simulink model "Quadcopter_nonlinear_LQIDG"  (R2020a)
settings: Solver=ode4  StartTime=0.0  StopTime=15  FixedStep=0.02  RelTol=1e-3
InitFcn:
  | Roll_OpenLoop_LQIDG_solver;
  | Pitch_OpenLoop_LQIDG_solver;
  | Yaw_OpenLoop_LQIDG_solver;
values from neighbouring files (symbols this model uses):
  A1 = 6.52172868745337    (= 6.52172868745)    [roll_pitch_yaw_parameter_estimation.m]
  A2 = -1.56517460219627    (= -1.5651746022)    [roll_pitch_yaw_parameter_estimation.m]
  A3 = 5.18692283683343e-05    (= 5.18692283683e-05)    [roll_pitch_yaw_parameter_estimation.m]
  A4 = 0.00249993776857667    (= 0.00249993776858)    [roll_pitch_yaw_parameter_estimation.m]
  A5 = -0.259645819519501    (= -0.25964581952)    [roll_pitch_yaw_parameter_estimation.m]
  A6 = 1.37409031322133    (= 1.37409031322)    [roll_pitch_yaw_parameter_estimation.m]
  B1 = 4.36026813860301    (= 4.3602681386)    [roll_pitch_yaw_parameter_estimation.m]
  B2 = 1.57068812881144    (= 1.57068812881)    [roll_pitch_yaw_parameter_estimation.m]
  B3 = 6.9083e-05    [roll_pitch_yaw_parameter_estimation.m]
  B4 = -0.00274841569825112    (= -0.00274841569825)    [roll_pitch_yaw_parameter_estimation.m]
  B5 = 0.595980110229882    (= 0.59598011023)    [roll_pitch_yaw_parameter_estimation.m]
  B6 = 4.42876359313229    (= 4.42876359313)    [roll_pitch_yaw_parameter_estimation.m]
  C1 = 0.0856557051952501    (= 0.0856557051953)    [roll_pitch_yaw_parameter_estimation.m]
  C2 = 1.26915503141054e-06    (= 1.26915503141e-06)    [roll_pitch_yaw_parameter_estimation.m]
  C3 = 0.178562738125068    (= 0.178562738125)    [roll_pitch_yaw_parameter_estimation.m]
  LQIDG_openloop_roll = (R1_inv * B' * p1)    [Roll_OpenLoop_LQIDG_solver.m]
undefined symbols (not defined in the file or in its folder): DiscIntNeverNeededParam, LQIDG_openloop_pitch, LQIDG_openloop_yaw, magnitude
libraries: simulink x1, simulink_extras x1
settings Model: Creator=Ali  LastModifiedBy=Ali

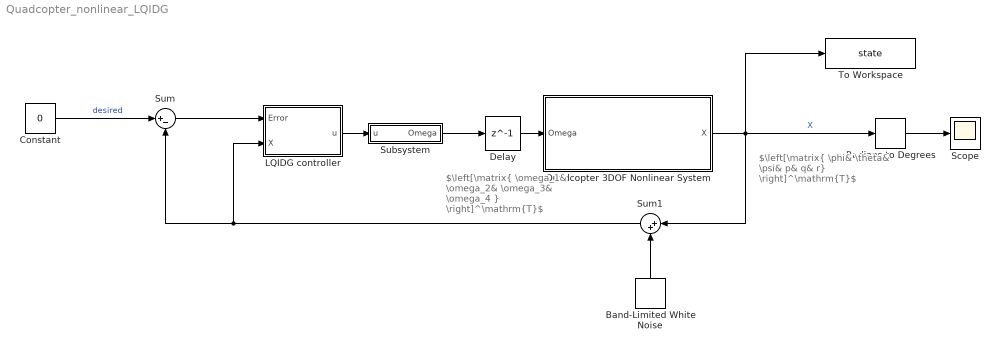
== system Quadcopter_nonlinear_LQIDG ==
  note: $\left[\matrix{ \omega_1& \omega_2& \omega_3& \omega_4 } \right]^\mathrm{T}$
  note: $\left[\matrix{ \phi& \theta& \psi& p& q& r} \right]^\mathrm{T}$
  Band-Limited White Noise : simulink/Sources/Band-Limited White Noise  Cov=[0.00001]  Ts=0.02  seed=[23341]
  Constant : Constant  Value=0
  Delay : Delay  DelayLength=1
  LQIDG controller : Subsystem
  Quadcopter 3DOF Nonlinear System : Subsystem  TreatAsAtomicUnit=on
      mask Display: image('quad1.png'); % Use "Edit Image" on toolstrip to change.
  Radians to Degrees : simulink_extras/Transformations/Radians to Degrees
  Scope : Scope
  Subsystem : Subsystem
  Sum : Sum  Inputs=|+-
  Sum1 : Sum  Inputs=|++
  To Workspace : ToWorkspace  VariableName=state  SampleTime=-1
  wires:
  Subsystem/1(Omega) -> Delay/1
  LQIDG controller/1(u) -> Subsystem/1(u)
  Sum/1 -> LQIDG controller/1(Error)
  Constant/1 -> Sum/1  "desired"
  Quadcopter 3DOF Nonlinear System/1(X) -> To Workspace/1, Sum1/1, Radians to Degrees/1  "X"
  Delay/1 -> Quadcopter 3DOF Nonlinear System/1(Omega)
  Radians to Degrees/1 -> Scope/1
  Sum1/1 -> LQIDG controller/2(X), Sum/2
  Band-Limited White Noise/1 -> Sum1/2

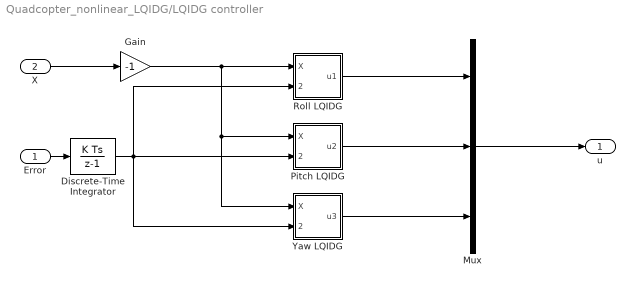
== system Quadcopter_nonlinear_LQIDG/LQIDG controller ==
  Error : Inport
  X : Inport  Port=2
  Discrete-Time Integrator : DiscreteIntegrator  SampleTime=-1  UpperSaturationLimit=2  LowerSaturationLimit=-2  ICPrevOutput=DiscIntNeverNeededParam  ICPrevScaledInput=DiscIntNeverNeededParam
  Gain : Gain  Gain=-1
  Mux : Mux  Inputs=3
  Pitch LQIDG : Subsystem
  Roll LQIDG : Subsystem
  Yaw LQIDG : Subsystem
  u : Outport
  wires:
  X/1 -> Gain/1
  Gain/1 -> Yaw LQIDG/1(X), Pitch LQIDG/1(X), Roll LQIDG/1(X)
  Error/1 -> Discrete-Time Integrator/1
  Roll LQIDG/1(u1) -> Mux/1
  Pitch LQIDG/1(u2) -> Mux/2
  Yaw LQIDG/1(u3) -> Mux/3
  Mux/1 -> u/1
  Discrete-Time Integrator/1 -> Roll LQIDG/2(Error), Yaw LQIDG/2(Error), Pitch LQIDG/2(Error)

== system Quadcopter_nonlinear_LQIDG/Quadcopter 3DOF Nonlinear System ==
  note: $\dot X$
  note: $\left[\matrix{ \dot\phi& \dot\theta& \dot\psi& \dot p& \dot q& \dot r} \right]^\mathrm{T}$
  note: $\left[\matrix{ \phi& \theta& \psi& p& q& r} \right]^\mathrm{T}$
  Omega : Inport
  Integrator : Integrator  InitialCondition=[-0.5, -1, 1, 0, 0, 0]
  Quad System : Subsystem
  Subsystem : Subsystem
  X : Outport
  wires:
  Integrator/1 -> Quad System/1(X), X/1  "X"
  Quad System/1(dot(X)) -> Integrator/1  "dot(X)"
  Omega/1 -> Subsystem/1(motor command)
  Subsystem/1(motor output) -> Quad System/2(Omega)

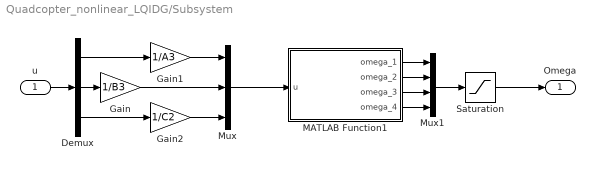
== system Quadcopter_nonlinear_LQIDG/Subsystem ==
  u : Inport
  Demux : Demux  Outputs=3
  Gain : Gain  Gain=1/B3
  Gain1 : Gain  Gain=1/A3
  Gain2 : Gain  Gain=1/C2
  MATLAB Function1 : MATLAB Function  TreatAsAtomicUnit=on
  Mux : Mux  Inputs=3
  Mux1 : Mux
  Saturation : Saturate  UpperLimit=6000/60*2*pi  LowerLimit=1300/60*2*pi
  Omega : Outport
  wires:
  MATLAB Function1/1(omega_1) -> Mux1/1
  MATLAB Function1/2(omega_2) -> Mux1/2
  MATLAB Function1/4(omega_4) -> Mux1/4
  MATLAB Function1/3(omega_3) -> Mux1/3
  Mux1/1 -> Saturation/1
  Mux/1 -> MATLAB Function1/1(u)
  Gain/1 -> Mux/2
  Gain1/1 -> Mux/1
  u/1 -> Demux/1
  Demux/2 -> Gain/1
  Demux/1 -> Gain1/1
  Demux/3 -> Gain2/1
  Gain2/1 -> Mux/3
  Saturation/1 -> Omega/1

== system Quadcopter_nonlinear_LQIDG/LQIDG controller/Pitch LQIDG ==
  X : Inport
  Error : Inport  Port=2
  Constant : Constant  Value=LQIDG_openloop_pitch
  Mux : Mux  Inputs=2
  Product : Product  Multiplication=Matrix(*)
  Selector : Selector  InputPortWidth=6  IndexOptions=Index vector (dialog)  Indices=[2 5]  OutputSizes=1
  Selector1 : Selector  InputPortWidth=6  IndexOptions=Index vector (dialog)  Indices=[2 5]  OutputSizes=1
  u2 : Outport
  wires:
  Product/1 -> u2/1
  Constant/1 -> Product/2
  Selector1/1 -> Mux/2
  Selector/1 -> Mux/1
  Error/1 -> Selector1/1
  X/1 -> Selector/1
  Mux/1 -> Product/1

== system Quadcopter_nonlinear_LQIDG/LQIDG controller/Roll LQIDG ==
  X : Inport
  Error : Inport  Port=2
  Constant : Constant  Value=LQIDG_openloop_roll
  Mux : Mux  Inputs=2
  Product : Product  Multiplication=Matrix(*)
  Selector : Selector  InputPortWidth=6  IndexOptions=Index vector (dialog)  Indices=[1 4]  OutputSizes=1
  Selector1 : Selector  InputPortWidth=6  IndexOptions=Index vector (dialog)  Indices=[1 4]  OutputSizes=1
  u1 : Outport
  wires:
  Product/1 -> u1/1
  Constant/1 -> Product/2
  X/1 -> Selector/1
  Error/1 -> Selector1/1
  Mux/1 -> Product/1
  Selector/1 -> Mux/1
  Selector1/1 -> Mux/2

== system Quadcopter_nonlinear_LQIDG/LQIDG controller/Yaw LQIDG ==
  X : Inport
  Error : Inport  Port=2
  Constant : Constant  Value=LQIDG_openloop_yaw
  Mux : Mux  Inputs=2
  Product : Product  Multiplication=Matrix(*)
  Selector : Selector  InputPortWidth=6  IndexOptions=Index vector (dialog)  Indices=[3 6]  OutputSizes=1
  Selector1 : Selector  InputPortWidth=6  IndexOptions=Index vector (dialog)  Indices=[3 6]  OutputSizes=1
  u3 : Outport
  wires:
  Product/1 -> u3/1
  Constant/1 -> Product/2
  Mux/1 -> Product/1
  Selector1/1 -> Mux/2
  Error/1 -> Selector1/1
  X/1 -> Selector/1
  Selector/1 -> Mux/1

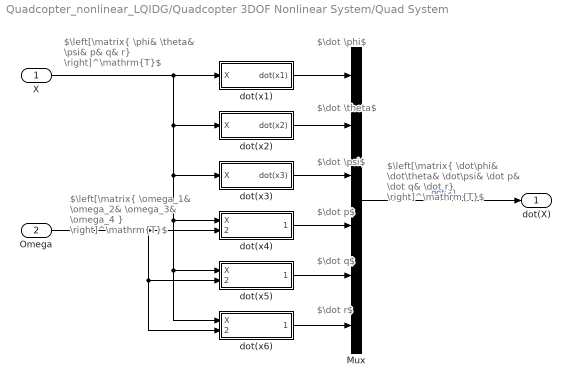
== system Quadcopter_nonlinear_LQIDG/Quadcopter 3DOF Nonlinear System/Quad System ==
  note: $\dot \phi$
  note: $\left[\matrix{ \phi& \theta& \psi& p& q& r} \right]^\mathrm{T}$
  note: $\left[\matrix{ \omega_1& \omega_2& \omega_3& \omega_4 } \right]^\mathrm{T}$
  note: $\dot \theta$
  note: $\dot \psi$
  note: $\dot p$
  note: $\dot q$
  note: $\dot r$
  note: $\left[\matrix{ \dot\phi& \dot\theta& \dot\psi& \dot p& \dot q& \dot r} \right]^\mathrm{T}$
  X : Inport
  Omega : Inport  Port=2
  Mux : Mux  Inputs=6
  dot(x1) : Subsystem
  dot(x2) : Subsystem
  dot(x3) : Subsystem
  dot(x4) : Subsystem
  dot(x5) : Subsystem
  dot(x6) : Subsystem
  dot(X) : Outport
  wires:
  Mux/1 -> dot(X)/1  "dot(X)"
  X/1 -> dot(x6)/1(X), dot(x5)/1(X), dot(x4)/1(X), dot(x3)/1(X), dot(x2)/1(X), dot(x1)/1(X)
  Omega/1 -> dot(x6)/2(Omega), dot(x5)/2(Omega), dot(x4)/2(Omega)
  dot(x5)/1(dot(x5)) -> Mux/5
  dot(x2)/1(dot(x2)) -> Mux/2
  dot(x4)/1(dot(x4)) -> Mux/4
  dot(x3)/1(dot(x3)) -> Mux/3
  dot(x1)/1(dot(x1)) -> Mux/1
  dot(x6)/1(dot(x6)) -> Mux/6

== system Quadcopter_nonlinear_LQIDG/Quadcopter 3DOF Nonlinear System/Subsystem ==
  motor command : Inport
  For Each Subsystem : Subsystem  TreatAsAtomicUnit=on
  motor output : Outport
  wires:
  motor command/1 -> For Each Subsystem/1(Omega_c)
  For Each Subsystem/1(Omega_m) -> motor output/1

== system Quadcopter_nonlinear_LQIDG/Quadcopter 3DOF Nonlinear System/Quad System/dot(x1) ==
  X : Inport
  1 : Subsystem
  Add : Sum  Inputs=+++
  Subsystem : Subsystem
  Subsystem1 : Subsystem
  dot(x1) : Outport
  wires:
  X/1 -> Subsystem1/1(X), Subsystem/1(X), 1/1(X)  "X"
  Subsystem1/1(x4) -> Add/3
  Subsystem/1(x6cos(x1)tan(x2)) -> Add/2
  Add/1 -> dot(x1)/1
  1/1(x5sin(x1)tan(x2)) -> Add/1

== system Quadcopter_nonlinear_LQIDG/Quadcopter 3DOF Nonlinear System/Quad System/dot(x2) ==
  X : Inport
  1 : Subsystem
  Add : Sum  Inputs=+-
  Subsystem : Subsystem
  dot(x2) : Outport
  wires:
  X/1 -> Subsystem/1(X), 1/1(X)  "X"
  Subsystem/1(x6sin(x1)) -> Add/2
  Add/1 -> dot(x2)/1
  1/1(x5cos(x1)) -> Add/1

== system Quadcopter_nonlinear_LQIDG/Quadcopter 3DOF Nonlinear System/Quad System/dot(x3) ==
  X : Inport
  1 : Subsystem
  Add : Sum
  Product : Product
  Subsystem : Subsystem
  Subsystem1 : Subsystem
  dot(x3) : Outport
  wires:
  X/1 -> Subsystem1/1(X), Subsystem/1(X), 1/1(X)  "X"
  Subsystem/1(x6cos(x1)) -> Add/2
  1/1(x5sin(x1)) -> Add/1
  Product/1 -> dot(x3)/1
  Add/1 -> Product/1
  Subsystem1/1(sec(x2)) -> Product/2

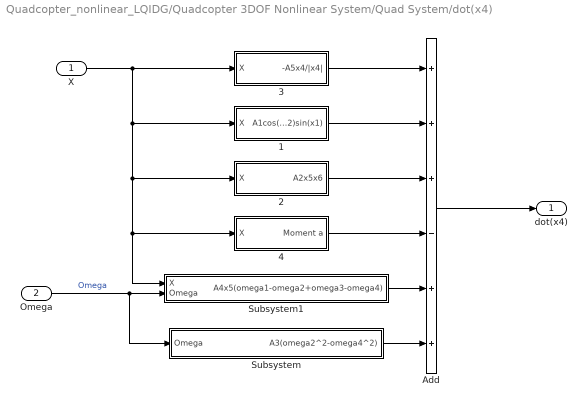
== system Quadcopter_nonlinear_LQIDG/Quadcopter 3DOF Nonlinear System/Quad System/dot(x4) ==
  X : Inport
  Omega : Inport  Port=2
  1 : Subsystem
  2 : Subsystem
  3 : Subsystem
  4 : Subsystem
  Add : Sum  Inputs=+++-++
  Subsystem : Subsystem
  Subsystem1 : Subsystem
  dot(x4) : Outport
  wires:
  X/1 -> 4/1(X), Subsystem1/1(X), 2/1(X), 1/1(X), 3/1(X)
  Omega/1 -> Subsystem/1(Omega), Subsystem1/2(Omega)  "Omega"
  Add/1 -> dot(x4)/1
  3/1("-A5x4/|x4| ") -> Add/1
  1/1(A1cos(x2)sin(x1)) -> Add/2
  2/1(A2x5x6) -> Add/3
  Subsystem1/1(A4x5(omega1-omega2+omega3-omega4)) -> Add/5
  Subsystem/1(A3(omega2^2-omega4^2)) -> Add/6
  4/1(Moment a) -> Add/4

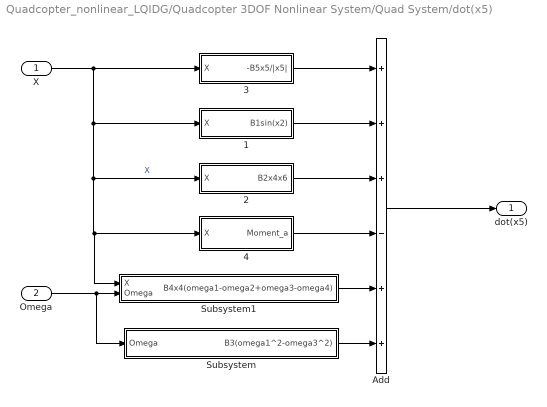
== system Quadcopter_nonlinear_LQIDG/Quadcopter 3DOF Nonlinear System/Quad System/dot(x5) ==
  X : Inport
  Omega : Inport  Port=2
  1 : Subsystem
  2 : Subsystem
  3 : Subsystem
  4 : Subsystem
  Add : Sum  Inputs=+++-++
  Subsystem : Subsystem
  Subsystem1 : Subsystem
  dot(x5) : Outport
  wires:
  Omega/1 -> Subsystem/1(Omega), Subsystem1/2(Omega)
  Add/1 -> dot(x5)/1
  3/1("-B5x5/|x5| ") -> Add/1
  1/1(B1sin(x2)) -> Add/2
  2/1(B2x4x6) -> Add/3
  Subsystem1/1(B4x4(omega1-omega2+omega3-omega4)) -> Add/5
  Subsystem/1(B3(omega1^2-omega3^2)) -> Add/6
  4/1(Moment_a) -> Add/4
  X/1 -> Subsystem1/1(X), 4/1(X), 2/1(X), 1/1(X), 3/1(X)  "X"

== system Quadcopter_nonlinear_LQIDG/Quadcopter 3DOF Nonlinear System/Quad System/dot(x6) ==
  X : Inport
  Omega : Inport  Port=2
  2 : Subsystem
  3 : Subsystem
  Add : Sum  Inputs=+++
  Subsystem : Subsystem
  dot(x6) : Outport
  wires:
  Omega/1 -> Subsystem/1(Omega)  "Omega"
  Add/1 -> dot(x6)/1
  3/1("-C3x6/|x6| ") -> Add/1
  2/1(C1x4x5) -> Add/2
  Subsystem/1(C2(omega1^2-omega2^2+omega3^2-omega4^2)) -> Add/3
  X/1 -> 2/1(X), 3/1(X)  "X"

== system Quadcopter_nonlinear_LQIDG/Quadcopter 3DOF Nonlinear System/Subsystem/For Each Subsystem ==
  Omega_c : Inport  Partition=on  PartitionDimension=1  PartitionWidth=1  PartitionOffset=0
  For Each : ForEach  DisableCoverage=on
  Transfer Fcn : TransferFcn  Denominator=[0.15 1]
  Omega_m : Outport  ConcatenationDimension=1
  wires:
  Omega_c/1 -> Transfer Fcn/1
  Transfer Fcn/1 -> Omega_m/1

== system Quadcopter_nonlinear_LQIDG/Quadcopter 3DOF Nonlinear System/Quad System/dot(x1)/1 ==
  X : Inport
  Demux : Demux  Outputs=6
  Subsystem : Subsystem
  Terminator : Terminator
  Terminator1 : Terminator
  Terminator2 : Terminator
  x5sin(x1)tan(x2) : Outport
  wires:
  Demux/2 -> Subsystem/2(x2)  "x2"
  Demux/4 -> Terminator1/1  "x4"
  X/1 -> Demux/1  "x"
  Demux/1 -> Subsystem/1(x1)  "x1"
  Demux/3 -> Terminator/1  "x3"
  Demux/6 -> Terminator2/1  "x6"
  Demux/5 -> Subsystem/3(x5)  "x5"
  Subsystem/1(x5sin(x1)tan(x2)) -> x5sin(x1)tan(x2)/1

== system Quadcopter_nonlinear_LQIDG/Quadcopter 3DOF Nonlinear System/Quad System/dot(x1)/Subsystem ==
  X : Inport
  Demux : Demux  Outputs=6
  Subsystem1 : Subsystem
  Terminator : Terminator
  Terminator1 : Terminator
  Terminator3 : Terminator
  x6cos(x1)tan(x2) : Outport
  wires:
  Demux/1 -> Subsystem1/1(x1)  "x1"
  Demux/3 -> Terminator/1  "x3"
  Demux/4 -> Terminator1/1  "x4"
  Demux/5 -> Terminator3/1  "x5"
  Demux/6 -> Subsystem1/3(x6)  "x6"
  Subsystem1/1(x6cos(x1)tan(x2)) -> x6cos(x1)tan(x2)/1  "x6cos(x1)tan(x2)"
  X/1 -> Demux/1  "X"
  Demux/2 -> Subsystem1/2(x2)  "x2"

== system Quadcopter_nonlinear_LQIDG/Quadcopter 3DOF Nonlinear System/Quad System/dot(x1)/Subsystem1 ==
  X : Inport
  Demux : Demux  Outputs=6
  Terminator{,2..5} (5 alike) : Terminator
  x4 : Outport
  wires:
  Demux/6 -> Terminator5/1  "x6"
  X/1 -> Demux/1
  Demux/3 -> Terminator/1  "x3"
  Demux/1 -> Terminator4/1  "x1"
  Demux/2 -> Terminator2/1  "x2"
  Demux/5 -> Terminator3/1  "x5"
  Demux/4 -> x4/1  "x4"

== system Quadcopter_nonlinear_LQIDG/Quadcopter 3DOF Nonlinear System/Quad System/dot(x2)/1 ==
  X : Inport
  Demux : Demux  Outputs=6
  Subsystem : Subsystem
  Terminator{,1..3} (4 alike) : Terminator
  x5cos(x1) : Outport
  wires:
  Demux/4 -> Terminator1/1  "x4"
  X/1 -> Demux/1  "x"
  Demux/1 -> Subsystem/1(x1)  "x1"
  Demux/3 -> Terminator/1  "x3"
  Demux/6 -> Terminator2/1  "x6"
  Demux/5 -> Subsystem/2(x5)  "x5"
  Subsystem/1(Out1) -> x5cos(x1)/1
  Demux/2 -> Terminator3/1  "x2"

== system Quadcopter_nonlinear_LQIDG/Quadcopter 3DOF Nonlinear System/Quad System/dot(x2)/Subsystem ==
  X : Inport
  Demux : Demux  Outputs=6
  Subsystem1 : Subsystem
  Terminator{,1..3} (4 alike) : Terminator
  x6sin(x1) : Outport
  wires:
  Demux/1 -> Subsystem1/1(x1)  "x1"
  Demux/3 -> Terminator/1  "x3"
  Demux/4 -> Terminator1/1  "x4"
  Demux/5 -> Terminator3/1  "x5"
  Demux/6 -> Subsystem1/2(x6)  "x6"
  Subsystem1/1(Out1) -> x6sin(x1)/1  "x6sin(x1)"
  X/1 -> Demux/1  "X"
  Demux/2 -> Terminator2/1  "x2"

== system Quadcopter_nonlinear_LQIDG/Quadcopter 3DOF Nonlinear System/Quad System/dot(x3)/1 ==
  X : Inport
  Demux : Demux  Outputs=6
  Subsystem : Subsystem
  Terminator{,1..3} (4 alike) : Terminator
  x5sin(x1) : Outport
  wires:
  Demux/4 -> Terminator1/1  "x4"
  X/1 -> Demux/1  "x"
  Demux/1 -> Subsystem/1(x1)  "x1"
  Demux/3 -> Terminator/1  "x3"
  Demux/6 -> Terminator2/1  "x6"
  Demux/5 -> Subsystem/2(x5)  "x5"
  Subsystem/1(x5sin(x1)) -> x5sin(x1)/1
  Demux/2 -> Terminator3/1  "x2"

== system Quadcopter_nonlinear_LQIDG/Quadcopter 3DOF Nonlinear System/Quad System/dot(x3)/Subsystem ==
  X : Inport
  Demux : Demux  Outputs=6
  Subsystem1 : Subsystem
  Terminator{,1..3} (4 alike) : Terminator
  x6cos(x1) : Outport
  wires:
  Demux/1 -> Subsystem1/1(x1)  "x1"
  Demux/3 -> Terminator/1  "x3"
  Demux/4 -> Terminator1/1  "x4"
  Demux/5 -> Terminator3/1  "x5"
  Demux/6 -> Subsystem1/2(x6)  "x6"
  Subsystem1/1(Out1) -> x6cos(x1)/1  "x6cos(x1)"
  X/1 -> Demux/1  "X"
  Demux/2 -> Terminator2/1  "x2"

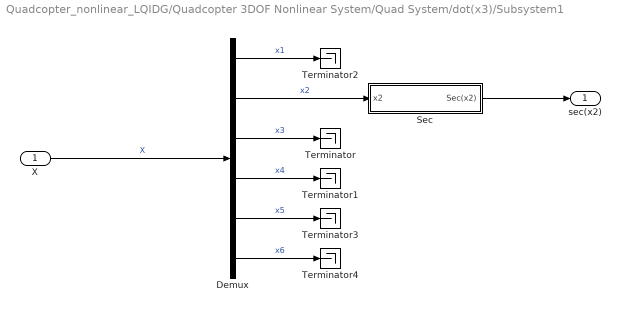
== system Quadcopter_nonlinear_LQIDG/Quadcopter 3DOF Nonlinear System/Quad System/dot(x3)/Subsystem1 ==
  X : Inport
  Demux : Demux  Outputs=6
  Sec : Subsystem
  Terminator{,1..4} (5 alike) : Terminator
  sec(x2) : Outport
  wires:
  Demux/3 -> Terminator/1  "x3"
  Demux/4 -> Terminator1/1  "x4"
  Demux/5 -> Terminator3/1  "x5"
  X/1 -> Demux/1  "X"
  Demux/1 -> Terminator2/1  "x1"
  Demux/6 -> Terminator4/1  "x6"
  Demux/2 -> Sec/1(x2)  "x2"
  Sec/1(Sec(x2)) -> sec(x2)/1

== system Quadcopter_nonlinear_LQIDG/Quadcopter 3DOF Nonlinear System/Quad System/dot(x4)/1 ==
  X : Inport
  Demux : Demux  Outputs=6
  Subsystem : Subsystem
  Terminator{,1..3} (4 alike) : Terminator
  A1cos(x2)sin(x1) : Outport
  wires:
  Demux/4 -> Terminator1/1  "x4"
  X/1 -> Demux/1  "x"
  Demux/1 -> Subsystem/1(x1)  "x1"
  Demux/3 -> Terminator/1  "x3"
  Demux/6 -> Terminator2/1  "x6"
  Subsystem/1(A1cos(x2)sin(x1)) -> A1cos(x2)sin(x1)/1
  Demux/2 -> Subsystem/2(x2)  "x2"
  Demux/5 -> Terminator3/1  "x5"

== system Quadcopter_nonlinear_LQIDG/Quadcopter 3DOF Nonlinear System/Quad System/dot(x4)/2 ==
  X : Inport
  Demux : Demux  Outputs=6
  Subsystem : Subsystem
  Terminator{,1,4..5} (4 alike) : Terminator
  A2x5x6 : Outport
  wires:
  Demux/4 -> Terminator1/1  "x4"
  X/1 -> Demux/1  "x"
  Demux/3 -> Terminator/1  "x3"
  Demux/6 -> Subsystem/2(x6)  "x6"
  Subsystem/1(A2x5x6) -> A2x5x6/1
  Demux/5 -> Subsystem/1(x5)  "x5"
  Demux/1 -> Terminator4/1  "x1"
  Demux/2 -> Terminator5/1  "x2"

== system Quadcopter_nonlinear_LQIDG/Quadcopter 3DOF Nonlinear System/Quad System/dot(x4)/3 ==
  X : Inport
  Demux : Demux  Outputs=6
  Subsystem : Subsystem
  Terminator{,2..5} (5 alike) : Terminator
  "-A5x4/|x4| " : Outport
  wires:
  X/1 -> Demux/1  "x"
  Demux/1 -> Terminator5/1  "x1"
  Demux/3 -> Terminator/1  "x3"
  Demux/6 -> Terminator2/1  "x6"
  Demux/2 -> Terminator4/1  "x2"
  Demux/5 -> Terminator3/1  "x5"
  Demux/4 -> Subsystem/1(x4)  "x4"
  Subsystem/1("-A5x4/|x4| ") -> "-A5x4/|x4| "/1

== system Quadcopter_nonlinear_LQIDG/Quadcopter 3DOF Nonlinear System/Quad System/dot(x4)/4 ==
  X : Inport
  Selector : Selector  InputPortWidth=6  IndexOptions=Index vector (dialog)  Indices=[1]  OutputSizes=1
  Subsystem : Subsystem
  Moment a : Outport
  wires:
  Selector/1 -> Subsystem/1(x1)  "x1"
  Subsystem/1(Moment_a) -> Moment a/1
  X/1 -> Selector/1  "x"

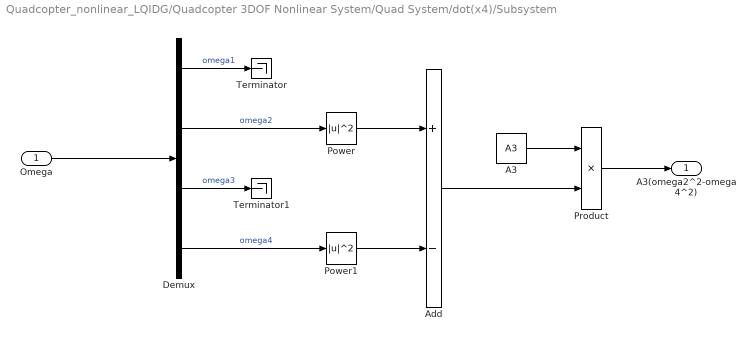
== system Quadcopter_nonlinear_LQIDG/Quadcopter 3DOF Nonlinear System/Quad System/dot(x4)/Subsystem ==
  Omega : Inport
  A3 : Constant  Value=A3
  Add : Sum  Inputs=+-
  Demux : Demux
  Power : Math  Operator=magnitude^2  SaturateOnIntegerOverflow=on
  Power1 : Math  Operator=magnitude^2  SaturateOnIntegerOverflow=on
  Product : Product
  Terminator : Terminator
  Terminator1 : Terminator
  A3(omega2^2-omega4^2) : Outport
  wires:
  Product/1 -> A3(omega2^2-omega4^2)/1
  Power1/1 -> Add/2
  Demux/2 -> Power/1  "omega2"
  Demux/4 -> Power1/1  "omega4"
  Add/1 -> Product/2
  Power/1 -> Add/1
  A3/1 -> Product/1
  Omega/1 -> Demux/1
  Demux/3 -> Terminator1/1  "omega3"
  Demux/1 -> Terminator/1  "omega1"

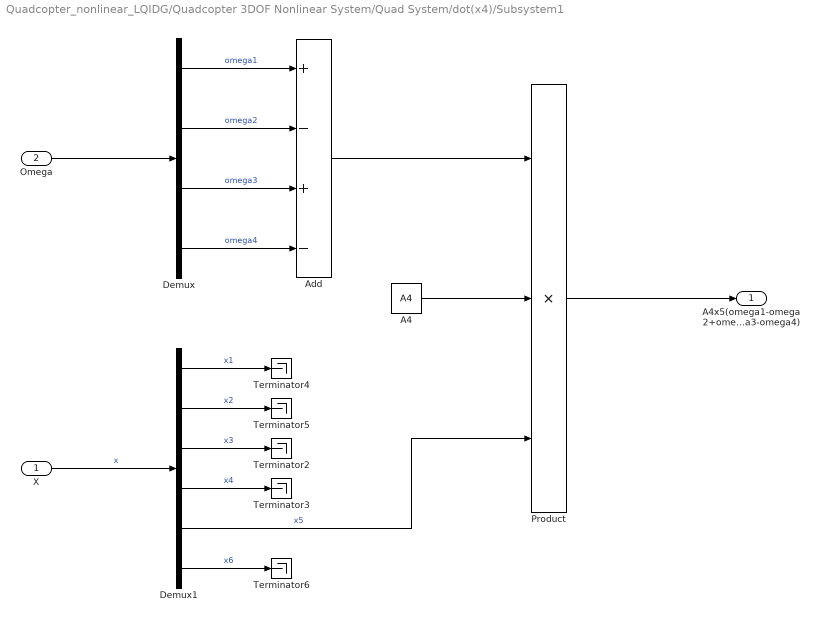
== system Quadcopter_nonlinear_LQIDG/Quadcopter 3DOF Nonlinear System/Quad System/dot(x4)/Subsystem1 ==
  X : Inport
  Omega : Inport  Port=2
  A4 : Constant  Value=A4
  Add : Sum  Inputs=+-+-
  Demux : Demux
  Demux1 : Demux  Outputs=6
  Product : Product  Inputs=3
  Terminator{2..6} (5 alike) : Terminator
  A4x5(omega1-omega2+omega3-omega4) : Outport
  wires:
  Omega/1 -> Demux/1
  Demux1/6 -> Terminator6/1  "x6"
  Demux1/5 -> Product/3  "x5"
  X/1 -> Demux1/1  "x"
  Demux1/2 -> Terminator5/1  "x2"
  Demux1/3 -> Terminator2/1  "x3"
  Demux1/4 -> Terminator3/1  "x4"
  Demux1/1 -> Terminator4/1  "x1"
  Demux/1 -> Add/1  "omega1"
  Demux/2 -> Add/2  "omega2"
  Demux/3 -> Add/3  "omega3"
  Demux/4 -> Add/4  "omega4"
  Add/1 -> Product/1
  A4/1 -> Product/2
  Product/1 -> A4x5(omega1-omega2+omega3-omega4)/1

== system Quadcopter_nonlinear_LQIDG/Quadcopter 3DOF Nonlinear System/Quad System/dot(x5)/1 ==
  X : Inport
  Demux : Demux  Outputs=6
  Subsystem : Subsystem
  Terminator{,1..4} (5 alike) : Terminator
  B1sin(x2) : Outport
  wires:
  Demux/4 -> Terminator1/1  "x4"
  X/1 -> Demux/1  "x"
  Demux/3 -> Terminator/1  "x3"
  Demux/6 -> Terminator2/1  "x6"
  Subsystem/1(B1sin(x2)) -> B1sin(x2)/1
  Demux/2 -> Subsystem/1(x2)  "x2"
  Demux/5 -> Terminator3/1  "x5"
  Demux/1 -> Terminator4/1  "x1"

== system Quadcopter_nonlinear_LQIDG/Quadcopter 3DOF Nonlinear System/Quad System/dot(x5)/2 ==
  X : Inport
  Demux : Demux  Outputs=6
  Subsystem : Subsystem
  Terminator{,2,4..5} (4 alike) : Terminator
  B2x4x6 : Outport
  wires:
  Demux/4 -> Subsystem/1(x4)  "x4"
  X/1 -> Demux/1  "x"
  Demux/3 -> Terminator/1  "x3"
  Demux/6 -> Subsystem/2(x6)  "x6"
  Subsystem/1(B2x4x6) -> B2x4x6/1
  Demux/1 -> Terminator4/1  "x1"
  Demux/2 -> Terminator5/1  "x2"
  Demux/5 -> Terminator2/1  "x5"

== system Quadcopter_nonlinear_LQIDG/Quadcopter 3DOF Nonlinear System/Quad System/dot(x5)/3 ==
  X : Inport
  Demux : Demux  Outputs=6
  Subsystem : Subsystem
  Terminator{,1..2,4..5} (5 alike) : Terminator
  "-B5x5/|x5| " : Outport
  wires:
  X/1 -> Demux/1  "x"
  Demux/1 -> Terminator5/1  "x1"
  Demux/3 -> Terminator/1  "x3"
  Demux/6 -> Terminator2/1  "x6"
  Demux/2 -> Terminator4/1  "x2"
  Demux/5 -> Subsystem/1(x5)  "x5"
  Subsystem/1("-B5x5/|x5| ") -> "-B5x5/|x5| "/1
  Demux/4 -> Terminator1/1  "x4"

== system Quadcopter_nonlinear_LQIDG/Quadcopter 3DOF Nonlinear System/Quad System/dot(x5)/4 ==
  X : Inport
  Selector : Selector  InputPortWidth=6  IndexOptions=Index vector (dialog)  Indices=[2]  OutputSizes=1
  Subsystem : Subsystem
  Moment_a : Outport
  wires:
  X/1 -> Selector/1  "x"
  Subsystem/1(moment_a) -> Moment_a/1
  Selector/1 -> Subsystem/1(In1)

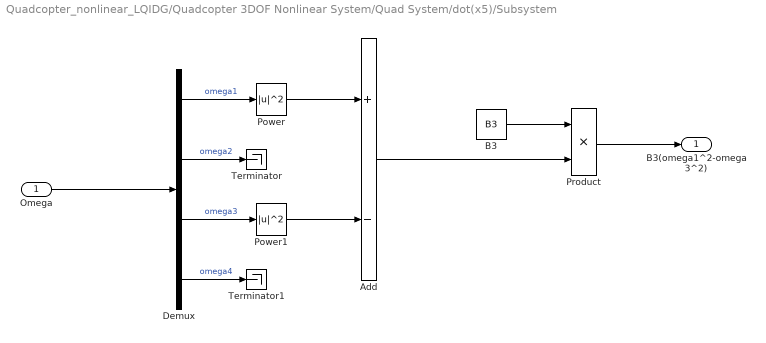
== system Quadcopter_nonlinear_LQIDG/Quadcopter 3DOF Nonlinear System/Quad System/dot(x5)/Subsystem ==
  Omega : Inport
  Add : Sum  Inputs=+-
  B3 : Constant  Value=B3
  Demux : Demux
  Power : Math  Operator=magnitude^2  SaturateOnIntegerOverflow=on
  Power1 : Math  Operator=magnitude^2  SaturateOnIntegerOverflow=on
  Product : Product
  Terminator : Terminator
  Terminator1 : Terminator
  B3(omega1^2-omega3^2) : Outport
  wires:
  Product/1 -> B3(omega1^2-omega3^2)/1
  Power1/1 -> Add/2
  Add/1 -> Product/2
  Power/1 -> Add/1
  B3/1 -> Product/1
  Omega/1 -> Demux/1
  Demux/3 -> Power1/1  "omega3"
  Demux/1 -> Power/1  "omega1"
  Demux/2 -> Terminator/1  "omega2"
  Demux/4 -> Terminator1/1  "omega4"

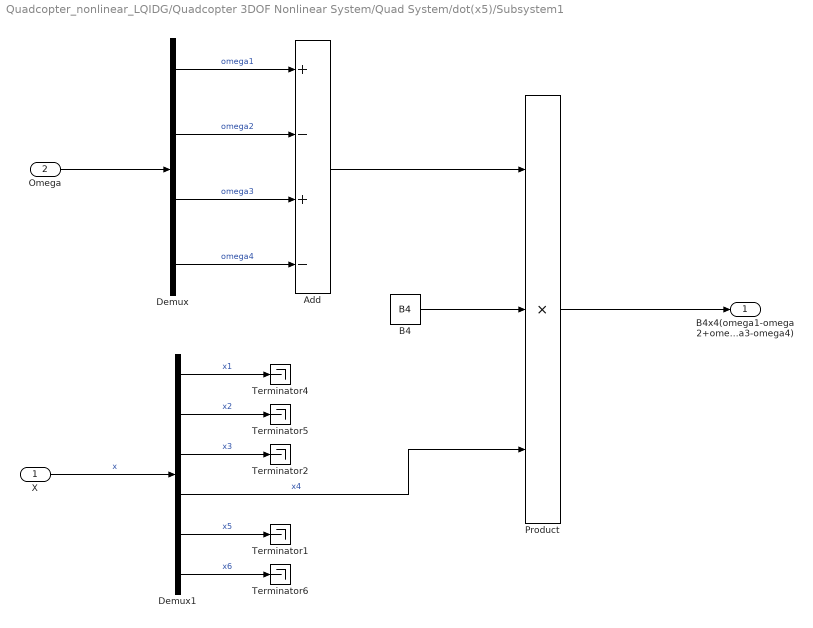
== system Quadcopter_nonlinear_LQIDG/Quadcopter 3DOF Nonlinear System/Quad System/dot(x5)/Subsystem1 ==
  X : Inport
  Omega : Inport  Port=2
  Add : Sum  Inputs=+-+-
  B4 : Constant  Value=B4
  Demux : Demux
  Demux1 : Demux  Outputs=6
  Product : Product  Inputs=3
  Terminator{1..2,4..6} (5 alike) : Terminator
  B4x4(omega1-omega2+omega3-omega4) : Outport
  wires:
  Omega/1 -> Demux/1
  Demux1/6 -> Terminator6/1  "x6"
  X/1 -> Demux1/1  "x"
  Demux1/2 -> Terminator5/1  "x2"
  Demux1/3 -> Terminator2/1  "x3"
  Demux1/4 -> Product/3  "x4"
  Demux1/1 -> Terminator4/1  "x1"
  Demux/1 -> Add/1  "omega1"
  Demux/2 -> Add/2  "omega2"
  Demux/3 -> Add/3  "omega3"
  Demux/4 -> Add/4  "omega4"
  Add/1 -> Product/1
  B4/1 -> Product/2
  Product/1 -> B4x4(omega1-omega2+omega3-omega4)/1
  Demux1/5 -> Terminator1/1  "x5"

== system Quadcopter_nonlinear_LQIDG/Quadcopter 3DOF Nonlinear System/Quad System/dot(x6)/2 ==
  X : Inport
  Demux : Demux  Outputs=6
  Subsystem : Subsystem
  Terminator{,2,4..5} (4 alike) : Terminator
  C1x4x5 : Outport
  wires:
  Demux/4 -> Subsystem/1(x4)  "x4"
  X/1 -> Demux/1  "x"
  Demux/3 -> Terminator/1  "x3"
  Subsystem/1(C1x4x5) -> C1x4x5/1
  Demux/1 -> Terminator4/1  "x1"
  Demux/2 -> Terminator5/1  "x2"
  Demux/5 -> Subsystem/2(x5)  "x5"
  Demux/6 -> Terminator2/1  "x6"

== system Quadcopter_nonlinear_LQIDG/Quadcopter 3DOF Nonlinear System/Quad System/dot(x6)/3 ==
  X : Inport
  Demux : Demux  Outputs=6
  Subsystem : Subsystem
  Terminator{,1,3..5} (5 alike) : Terminator
  "-C3x6/|x6| " : Outport
  wires:
  X/1 -> Demux/1  "x"
  Demux/1 -> Terminator5/1  "x1"
  Demux/3 -> Terminator/1  "x3"
  Demux/6 -> Subsystem/1(x6)  "x6"
  Demux/2 -> Terminator4/1  "x2"
  Demux/5 -> Terminator3/1  "x5"
  Subsystem/1("-C3x6/|x6| ") -> "-C3x6/|x6| "/1
  Demux/4 -> Terminator1/1  "x4"

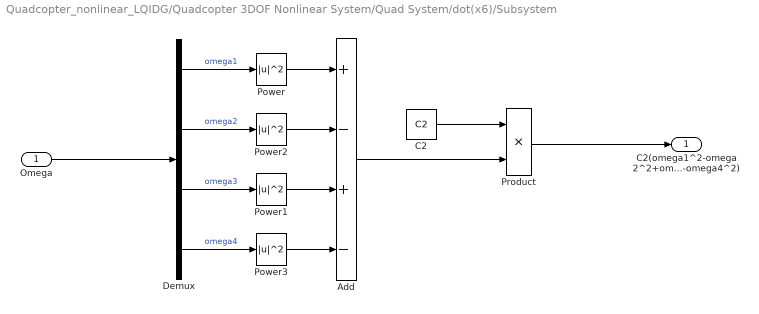
== system Quadcopter_nonlinear_LQIDG/Quadcopter 3DOF Nonlinear System/Quad System/dot(x6)/Subsystem ==
  Omega : Inport
  Add : Sum  Inputs=+-+-
  C2 : Constant  Value=C2
  Demux : Demux
  Power{,1..3} (4 alike) : Math  Operator=magnitude^2  SaturateOnIntegerOverflow=on
  Product : Product
  C2(omega1^2-omega2^2+omega3^2-omega4^2) : Outport
  wires:
  Omega/1 -> Demux/1
  Demux/3 -> Power1/1  "omega3"
  Demux/1 -> Power/1  "omega1"
  Demux/2 -> Power2/1  "omega2"
  Demux/4 -> Power3/1  "omega4"
  C2/1 -> Product/1
  Add/1 -> Product/2
  Product/1 -> C2(omega1^2-omega2^2+omega3^2-omega4^2)/1
  Power/1 -> Add/1
  Power2/1 -> Add/2
  Power1/1 -> Add/3
  Power3/1 -> Add/4

== system Quadcopter_nonlinear_LQIDG/Quadcopter 3DOF Nonlinear System/Quad System/dot(x1)/1/Subsystem ==
  x1 : Inport
  x2 : Inport  Port=2
  x5 : Inport  Port=3
  Product : Product  Inputs=3
  Sin : Trigonometry
  Tan : Trigonometry  Operator=tan
  x5sin(x1)tan(x2) : Outport
  wires:
  Sin/1 -> Product/1
  x5/1 -> Product/3
  Product/1 -> x5sin(x1)tan(x2)/1
  x1/1 -> Sin/1
  x2/1 -> Tan/1
  Tan/1 -> Product/2

== system Quadcopter_nonlinear_LQIDG/Quadcopter 3DOF Nonlinear System/Quad System/dot(x1)/Subsystem/Subsystem1 ==
  x1 : Inport
  x2 : Inport  Port=2
  x6 : Inport  Port=3
  Cos : Trigonometry  Operator=cos
  Product1 : Product  Inputs=3
  Tan : Trigonometry  Operator=tan
  x6cos(x1)tan(x2) : Outport
  wires:
  x6/1 -> Product1/3
  x1/1 -> Cos/1
  Cos/1 -> Product1/1
  x2/1 -> Tan/1
  Product1/1 -> x6cos(x1)tan(x2)/1
  Tan/1 -> Product1/2

== system Quadcopter_nonlinear_LQIDG/Quadcopter 3DOF Nonlinear System/Quad System/dot(x2)/1/Subsystem ==
  x1 : Inport
  x5 : Inport  Port=2
  Cos : Trigonometry  Operator=cos
  Product : Product
  Out1 : Outport
  wires:
  Cos/1 -> Product/1
  Product/1 -> Out1/1
  x1/1 -> Cos/1
  x5/1 -> Product/2

== system Quadcopter_nonlinear_LQIDG/Quadcopter 3DOF Nonlinear System/Quad System/dot(x2)/Subsystem/Subsystem1 ==
  x1 : Inport
  x6 : Inport  Port=2
  Product1 : Product
  Sin : Trigonometry
  Out1 : Outport
  wires:
  x6/1 -> Product1/2
  x1/1 -> Sin/1
  Sin/1 -> Product1/1
  Product1/1 -> Out1/1

== system Quadcopter_nonlinear_LQIDG/Quadcopter 3DOF Nonlinear System/Quad System/dot(x3)/1/Subsystem ==
  x1 : Inport
  x5 : Inport  Port=2
  Product : Product
  Sin : Trigonometry
  x5sin(x1) : Outport
  wires:
  Sin/1 -> Product/1
  Product/1 -> x5sin(x1)/1
  x1/1 -> Sin/1
  x5/1 -> Product/2

== system Quadcopter_nonlinear_LQIDG/Quadcopter 3DOF Nonlinear System/Quad System/dot(x3)/Subsystem/Subsystem1 ==
  x1 : Inport
  x6 : Inport  Port=2
  Cos : Trigonometry  Operator=cos
  Product1 : Product
  Out1 : Outport
  wires:
  x6/1 -> Product1/2
  x1/1 -> Cos/1
  Cos/1 -> Product1/1
  Product1/1 -> Out1/1

== system Quadcopter_nonlinear_LQIDG/Quadcopter 3DOF Nonlinear System/Quad System/dot(x3)/Subsystem1/Sec ==
  x2 : Inport
  Constant : Constant
  Cos : Trigonometry  Operator=cos
  Divide : Product  Inputs=*/
  Sec(x2) : Outport
  wires:
  Constant/1 -> Divide/1
  Cos/1 -> Divide/2
  Divide/1 -> Sec(x2)/1
  x2/1 -> Cos/1

== system Quadcopter_nonlinear_LQIDG/Quadcopter 3DOF Nonlinear System/Quad System/dot(x4)/1/Subsystem ==
  x1 : Inport
  x2 : Inport  Port=2
  A1 : Constant  Value=A1
  Cos : Trigonometry  Operator=cos
  Product : Product  Inputs=3
  Sin : Trigonometry
  A1cos(x2)sin(x1) : Outport
  wires:
  Sin/1 -> Product/1
  Product/1 -> A1cos(x2)sin(x1)/1
  x1/1 -> Sin/1
  x2/1 -> Cos/1
  Cos/1 -> Product/2
  A1/1 -> Product/3

== system Quadcopter_nonlinear_LQIDG/Quadcopter 3DOF Nonlinear System/Quad System/dot(x4)/2/Subsystem ==
  x5 : Inport
  x6 : Inport  Port=2
  A2 : Constant  Value=A2
  Product : Product  Inputs=3
  A2x5x6 : Outport
  wires:
  x5/1 -> Product/1
  Product/1 -> A2x5x6/1
  x6/1 -> Product/2
  A2/1 -> Product/3

== system Quadcopter_nonlinear_LQIDG/Quadcopter 3DOF Nonlinear System/Quad System/dot(x4)/3/Subsystem ==
  x4 : Inport
  A5 : Constant  Value=A5
  Gain : Gain  Gain=-1
  Switch : Switch  Criteria=u2 > Threshold
  "-A5x4/|x4| " : Outport
  wires:
  Switch/1 -> "-A5x4/|x4| "/1
  A5/1 -> Switch/3, Gain/1
  x4/1 -> Switch/2
  Gain/1 -> Switch/1

== system Quadcopter_nonlinear_LQIDG/Quadcopter 3DOF Nonlinear System/Quad System/dot(x4)/4/Subsystem ==
  x1 : Inport
  Aa : Constant  Value=A6
  Product : Product
  Sin : Trigonometry  Operator=cos
  Moment_a : Outport
  wires:
  Sin/1 -> Product/1
  Product/1 -> Moment_a/1
  x1/1 -> Sin/1
  Aa/1 -> Product/2

== system Quadcopter_nonlinear_LQIDG/Quadcopter 3DOF Nonlinear System/Quad System/dot(x5)/1/Subsystem ==
  x2 : Inport
  B1 : Constant  Value=B1
  Product : Product
  Sin : Trigonometry
  B1sin(x2) : Outport
  wires:
  Product/1 -> B1sin(x2)/1
  x2/1 -> Sin/1
  B1/1 -> Product/2
  Sin/1 -> Product/1

== system Quadcopter_nonlinear_LQIDG/Quadcopter 3DOF Nonlinear System/Quad System/dot(x5)/2/Subsystem ==
  x4 : Inport
  x6 : Inport  Port=2
  B2 : Constant  Value=B2
  Product : Product  Inputs=3
  B2x4x6 : Outport
  wires:
  x4/1 -> Product/1
  Product/1 -> B2x4x6/1
  x6/1 -> Product/2
  B2/1 -> Product/3

== system Quadcopter_nonlinear_LQIDG/Quadcopter 3DOF Nonlinear System/Quad System/dot(x5)/3/Subsystem ==
  x5 : Inport
  B5 : Constant  Value=B5
  Gain : Gain  Gain=-1
  Switch : Switch  Criteria=u2 > Threshold
  "-B5x5/|x5| " : Outport
  wires:
  Switch/1 -> "-B5x5/|x5| "/1
  B5/1 -> Switch/3, Gain/1
  x5/1 -> Switch/2
  Gain/1 -> Switch/1

== system Quadcopter_nonlinear_LQIDG/Quadcopter 3DOF Nonlinear System/Quad System/dot(x5)/4/Subsystem ==
  In1 : Inport
  Ba : Constant  Value=B6
  Cos : Trigonometry  Operator=cos
  Product : Product
  moment_a : Outport
  wires:
  Product/1 -> moment_a/1
  Ba/1 -> Product/1
  In1/1 -> Cos/1
  Cos/1 -> Product/2

== system Quadcopter_nonlinear_LQIDG/Quadcopter 3DOF Nonlinear System/Quad System/dot(x6)/2/Subsystem ==
  x4 : Inport
  x5 : Inport  Port=2
  C1 : Constant  Value=C1
  Product : Product  Inputs=3
  C1x4x5 : Outport
  wires:
  x4/1 -> Product/1
  Product/1 -> C1x4x5/1
  x5/1 -> Product/2
  C1/1 -> Product/3

== system Quadcopter_nonlinear_LQIDG/Quadcopter 3DOF Nonlinear System/Quad System/dot(x6)/3/Subsystem ==
  x6 : Inport
  C3 : Constant  Value=C3
  Gain : Gain  Gain=-1
  Switch : Switch  Criteria=u2 > Threshold
  "-C3x6/|x6| " : Outport
  wires:
  Switch/1 -> "-C3x6/|x6| "/1
  C3/1 -> Switch/3, Gain/1
  x6/1 -> Switch/2
  Gain/1 -> Switch/1

== matlab function Quadcopter_nonlinear_LQIDG/Subsystem/MATLAB Function1 ==
  data: u input size=3; omega_1 output size=1; omega_2 output size=1; omega_3 output size=1; omega_4 output size=1
function [omega_1, omega_2, omega_3, omega_4] = fcn(u)
u1 = u(1);
u2 = u(2);
u3 = u(3);
% control effort
u4 = ones(1, length(u1)) * 4 * rpm2rad_sec(3500)^2;
% calculate omega
if (u4 + u3 + 2 * u2) / 4 > 0
    omega_1 = sqrt((u4 + u3 + 2 * u2) / 4);
else
    omega_1 = 0;
end
if (u4 + u3 - 2 * u2) / 4 > 0
    omega_3 = sqrt((u4 + u3 - 2 * u2) / 4);
else
    omega_3 = 0;
end
if (u4 - u3 + 2 * u1) / 4 > 0
    omega_2 = sqrt((u4 - u3 + 2 * u1) / 4);
else
    omega_2 = 0;
end
if (u4 - u3 - 2 * u1) / 4 > 0
    omega_4 = sqrt((u4 - u3 - 2 * u1) / 4);
else
    omega_4 = 0;
end
end
%% functions
% rpm to rad/sec
function rad = rpm2rad_sec(rpm)
rad = rpm / 60 * 2 * pi;
end
